simulink model "ClosedLoopControl"  (R2016b)
settings: Solver=FixedStepDiscrete  StartTime=0.0  StopTime=Inf  FixedStep=sCoreParams.core.stepPeriod  RelTol=1e-3  EnableMultiTasking=on
undefined symbols (not defined in the file): fdesignblkfcn, gcbh, High, sCoreParams, sCoreParams_decoders_chanceDetector_randStimEventsPerSec, sCoreParams_decoders_txDetector_channel1, sCoreParams_decoders_txDetector_channel2, sCoreParams_decoders_txDetector_detectChannelInds, sCoreParams_decoders_txDetector_nChannels, sCoreParams_Features_Baseline_initialThresholdValue, sCoreParams_Features_Baseline_weightPreviousThreshold, sCoreParams_Features_Data_SmoothWindowsDurationSamples, sCoreParams_stimulator_stimAfterDelaySteps
libraries: dsparch4 x20, dspstat3 x19, dspspect3 x6, dspfdesign x2, dspindex x2, dspswit3 x1
(part 1 of 6)
settings Model: DataTypeOverride=Double  MinMaxOverflowLogging=ForceOff  Creator=rzelmann  LastModifiedBy=rzelmann
settings SolverCC: EnableConcurrentExecution=on  ConcurrentTasks=on
settings DataIOCC: SaveFormat=StructureWithTime  DSMLogging=off  SignalLoggingName=logsClosedLoopControl
settings OptimizationCC: DefaultParameterBehavior=Inlined  EfficientFloat2IntCast=on  LifeSpan=inf
settings DebuggingCC: AllowSymbolicDim=off  SFUnexpectedBacktrackingDiag=warning  SFNoUnconditionalDefaultTransitionDiag=warning  SFExecutionAtInitializationDiag=none
settings HardwareCC: ProdBitPerPointer=32  ProdBitPerSizeT=32  ProdBitPerPtrDiffT=32  ProdLargestAtomicFloat=None  ProdWordSize=32  ProdLongLongMode=on  ProdHWDeviceType=Generic->32-bit x86 compatible
settings ModelReferenceCC: UpdateModelReferenceTargets=Force  EnableParallelModelReferenceBuilds=on  ParallelModelReferenceMATLABWorkerInit=Copy Base Workspace  ModelReferenceNumInstancesAllowed=Single  ModelReferencePassRootInputsByReference=off
settings RTWCC: SystemTargetFile=slrt.tlc  TemplateMakefile=slrt_default_tmf  Description=Simulink Real-Time  RTWCompilerOptimization=on
settings CodeAppCC: MaxIdLength=63
settings ConfigComp: CovMetricSettings=dw  CovHtmlReporting=on  CovSaveCumulativeToWorkspaceVar=on  CovSaveSingleToWorkspaceVar=on  CovExternalEMLEnable=off

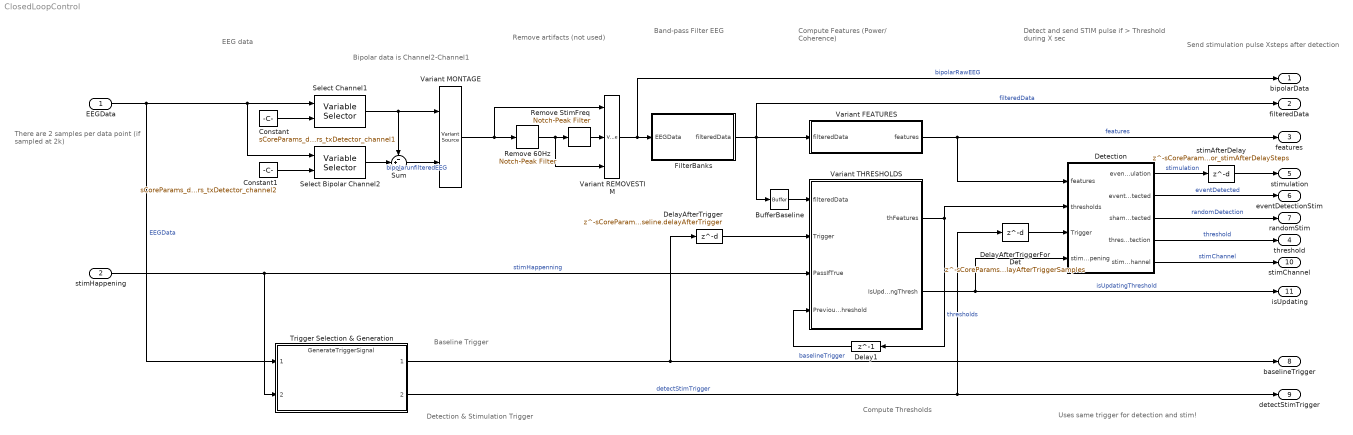
== system ClosedLoopControl ==
  note: Send stimulation pulse Xsteps after detection
  note: Bipolar data is Channel2-Channel1
  note: Baseline Trigger
  note: EEG data
  note: Uses same trigger for detection and stim!
  note: There are 2 samples per data point
      | (if sampled at 2k)
  note: Detection & Stimulation Trigger
  note: Band-pass
      | Filter EEG
  note: Compute Features
      | (Power/ Coherence)
  note: Remove artifacts
      | (not used)
  note: Detect and send STIM pulse
      | if > Threshold during X sec
  note: Compute Thresholds
  EEGData : Inport  OutDataTypeStr=double  PortDimensions=[sCoreParams.core.samplesPerStep sCoreParams.core.maxChannelsAllNSPs]  SampleTime=sCoreParams.core.stepPeriod
  stimHappening : Inport  Port=2  OutDataTypeStr=boolean  PortDimensions=1  SampleTime=sCoreParams.core.stepPeriod
  BufferBaseline : Buffer  N=sCoreParams.Features.Baseline.durationSamples  V=sCoreParams.Features.Baseline.durationSamples-sCoreParams.FrameSize  TreatMby1Signals=One channel  OutputFrames=off
  Constant : Constant  Value=sCoreParams_decoders_txDetector_channel1  SampleTime=Inf
  Constant1 : Constant  Value=sCoreParams_decoders_txDetector_channel2
  Delay1 : Delay  DelayLength=1  InitialCondition=sCoreParams_Features_Baseline_initialThresholdValue  InputProcessing=Inherited  SampleTime=sCoreParams.core.stepPeriod
  DelayAfterTrigger : Delay  DelayLength=sCoreParams.Features.Baseline.delayAfterTrigger  InitialCondition=sCoreParams.Features.Baseline.beforeFirstTrigger  InputProcessing=Columns as channels (frame based)  SampleTime=sCoreParams.core.stepPeriod
  DelayAfterTriggerForDet : Delay  DelayLength=sCoreParams.decoders.txDetector.delayAfterTriggerSamples  InitialCondition=0  InputProcessing=Columns as channels (frame based)  SampleTime=sCoreParams.core.stepPeriod
  Detection : Subsystem
  FilterBanks : Subsystem
  Remove 60Hz : dspfdesign/Notch-Peak Filter  Specification=Bandwidth and center frequency  Bandwidth=2  QualityFactor=5  CenterFrequency=60  BandwidthCoefficient=0.72654  CenterFrequencyCoefficient=0  Output=Notch  InheritSampleRate=off  SampleRate=sCoreParams.core.samplingRate  SimulateUsing=Code generation
  Remove StimFreq : dspfdesign/Notch-Peak Filter  Specification=Bandwidth and center frequency  Bandwidth=2  QualityFactor=5  CenterFrequency=sCoreParams_stimulationFrequencyHz  BandwidthCoefficient=0.72654  CenterFrequencyCoefficient=0  Output=Notch  InheritSampleRate=off  SampleRate=sCoreParams.core.samplingRate  SimulateUsing=Code generation
  Select Bipolar Channel2 : dspindex/Variable Selector  NumInputs=1  rowsOrCols=Columns  IdxMode=Variable  Elements=sCoreParams_decoders_txDetector_channel2  ZerOneIdxMode=One-based  errmode=Clip Index  FillMode=off  FillValues=0
  Select Channel1 : dspindex/Variable Selector  NumInputs=1  rowsOrCols=Columns  IdxMode=Variable  Elements=sCoreParams_decoders_txDetector_channel1  ZerOneIdxMode=One-based  errmode=Clip Index  FillMode=off  FillValues=0
  Sum : Sum  Inputs=-+|  InputSameDT=on
  Trigger Selection & Generation : ModelReference  ModelNameDialog=GenerateTriggerSignal  SimulationMode=Normal  ModelReferenceVersion=1.53
  Variant FEATURES : Subsystem  Variant=on
  Variant MONTAGE : VariantSource  Description=|
      | Variant MONTAGE allows to select between referential and bipolar montages,
      | Output is N referential or bipolar channels.
      | channel numbers are specified in variables:
      |  - sCoreParams.decoders.txDetector.channel1 
      |  - sCoreParams.decoders.txDetector.channel2
      | 
      | In the case of referential only sCoreParams.decoders.txDetector.channel1 is considered
  Variant REMOVESTIM : VariantSource  Description=|
      | Variant MONTAGE allows to select between referential and bipolar montages,
      | Output is N referential or bipolar channels.
      | channel numbers are specified in variables:
      |  - sCoreParams.decoders.txDetector.channel1 
      |  - sCoreParams.decoders.txDetector.channel2
      | 
      | In the case of referential only sCoreParams.decoders.txDetector.channel1 is considered
  Variant THRESHOLDS : Subsystem  Variant=on
  stimAfterDelay : Delay  DelayLength=sCoreParams_stimulator_stimAfterDelaySteps  InitialCondition=0  InputProcessing=Columns as channels (frame based)  SampleTime=sCoreParams.core.stepPeriod
  bipolarData : Outport
  filteredData : Outport  Port=2
  features : Outport  Port=3  SampleTime=sCoreParams.core.stepPeriod  BusOutputAsStruct=on
  threshold : Outport  Port=4
  stimulation : Outport  Port=5
  eventDetectionStim : Outport  Port=6
  randomStim : Outport  Port=7  OutDataTypeStr=boolean
  baselineTrigger : Outport  Port=8
  detectStimTrigger : Outport  Port=9
  stimChannel : Outport  Port=10  OutDataTypeStr=int32  PortDimensions=[1 2]
  isUpdating : Outport  Port=11
  wires:
  Detection/4(thresholdUsedInDetection) -> threshold/1  "threshold"
  Variant MONTAGE/1 -> Variant REMOVESTIM/1, Remove 60Hz/1
  Variant THRESHOLDS/2(IsUpdatingThresh) -> Detection/4(stimHappening), isUpdating/1  "isUpdatingThreshold"
  Select Channel1/1 -> Variant MONTAGE/1, Sum/1
  Sum/1 -> Variant MONTAGE/2  "bipolarunfilteredEEG"
  Select Bipolar Channel2/1 -> Sum/2
  Trigger Selection & Generation/1 -> DelayAfterTrigger/1, baselineTrigger/1  "baselineTrigger"
  Remove 60Hz/1 -> Variant REMOVESTIM/3, Remove StimFreq/1
  Variant REMOVESTIM/1 -> FilterBanks/1(EEGData), bipolarData/1  "bipolarRawEEG"
  stimHappening/1 -> Trigger Selection & Generation/2, Variant THRESHOLDS/3(PassIfTrue)  "stimHappenning"
  Constant/1 -> Select Channel1/2
  Constant1/1 -> Select Bipolar Channel2/2
  BufferBaseline/1 -> Variant THRESHOLDS/1(filteredData)
  Variant FEATURES/1(features) -> Detection/1(features), features/1  "features"
  Variant THRESHOLDS/1(thFeatures) -> Delay1/1, Detection/2(thresholds)  "thresholds"
  Delay1/1 -> Variant THRESHOLDS/4(PreviousThreshold)
  DelayAfterTrigger/1 -> Variant THRESHOLDS/2(Trigger)
  Trigger Selection & Generation/2 -> DelayAfterTriggerForDet/1, detectStimTrigger/1  "detectStimTrigger"
  DelayAfterTriggerForDet/1 -> Detection/3(Trigger)
  Detection/5(stimChannel) -> stimChannel/1  "stimChannel"
  EEGData/1 -> Select Bipolar Channel2/1, Select Channel1/1, Trigger Selection & Generation/1  "EEGData"
  Remove StimFreq/1 -> Variant REMOVESTIM/2
  FilterBanks/1(filteredData) -> BufferBaseline/1, filteredData/1, Variant FEATURES/1(filteredData)  "filteredData"
  Detection/3(shamDetected) -> randomStim/1  "randomDetection"
  Detection/2(eventDetected) -> eventDetectionStim/1  "eventDetected"
  Detection/1(eventStimulation) -> stimAfterDelay/1  "stimulation"
  stimAfterDelay/1 -> stimulation/1

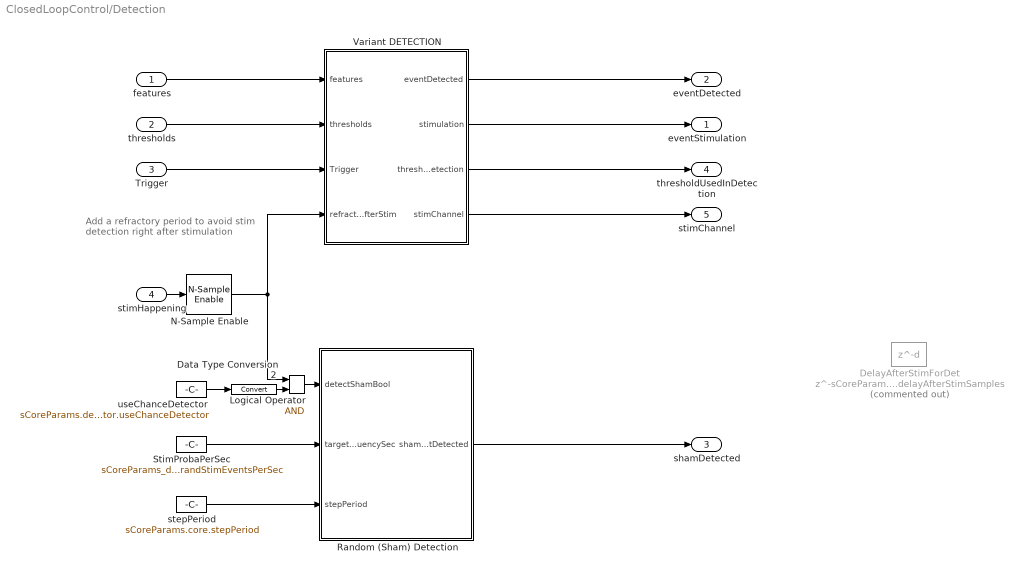
== system ClosedLoopControl/Detection ==
  note: Add a refractory period to avoid
      | stim detection right after stimulation
  features : Inport
  thresholds : Inport  Port=2
  Trigger : Inport  Port=3
  stimHappening : Inport  Port=4
  Data Type Conversion2 : DataTypeConversion
  DelayAfterStimForDet : Delay  Commented=on  DelayLength=sCoreParams.decoders.txDetector.delayAfterStimSamples  InitialCondition=0  InputProcessing=Columns as channels (frame based)  SampleTime=sCoreParams.core.stepPeriod
  Logical Operator : Logic  IconShape=distinctive  AllPortsSameDT=off  OutDataTypeStr=boolean
  N-Sample Enable : dspswit3/N-Sample Enable  N=sCoreParams.decoders.txDetector.delayAfterStimSteps  ActiveLevel=High (1)  reset=on  TriggerType=Rising edge  Ts=1  DataType=Logical
  Random (Sham) Detection : MATLAB Function  TreatAsAtomicUnit=on  SystemSampleTime=sCoreParams.core.stepPeriod
  StimProbaPerSec : Constant  Value=sCoreParams_decoders_chanceDetector_randStimEventsPerSec
  Variant DETECTION : Subsystem  Variant=on
  stepPeriod : Constant  Value=sCoreParams.core.stepPeriod
  useChanceDetector : Constant  Value=sCoreParams.decoders.chanceDetector.useChanceDetector
  eventStimulation : Outport
  eventDetected : Outport  Port=2
  shamDetected : Outport  Port=3  OutDataTypeStr=boolean
  thresholdUsedInDetection : Outport  Port=4
  stimChannel : Outport  Port=5
  wires:
  Variant DETECTION/2(stimulation) -> eventStimulation/1
  features/1 -> Variant DETECTION/1(features)
  thresholds/1 -> Variant DETECTION/2(thresholds)
  Trigger/1 -> Variant DETECTION/3(Trigger)
  Variant DETECTION/3(thresholdUsedInDetection) -> thresholdUsedInDetection/1
  Variant DETECTION/4(stimChannel) -> stimChannel/1
  stepPeriod/1 -> Random (Sham) Detection/3(stepPeriod)
  StimProbaPerSec/1 -> Random (Sham) Detection/2(targetShamFrequencySec)
  Logical Operator/1 -> Random (Sham) Detection/1(detectShamBool)
  Random (Sham) Detection/1(shamEventDetected) -> shamDetected/1
  Variant DETECTION/1(eventDetected) -> eventDetected/1
  stimHappening/1 -> N-Sample Enable/1
  N-Sample Enable/1 -> Logical Operator/1, Variant DETECTION/4(refractoryTimeAfterStim)
  useChanceDetector/1 -> Data Type Conversion2/1
  Data Type Conversion2/1 -> Logical Operator/2

== system ClosedLoopControl/FilterBanks ==
  note: Frequency band of the filter is FIXED in Simulink Real-Time
      | Add a new variant block if other sampling rates are required
  EEGData : Inport
  Variant FILTER 1000 : Subsystem  Variant=on
  Variant FILTER 2000 : Subsystem  Variant=on
  Variant SAMPLING RATE : VariantSource  Description=|
      | Variant MONTAGE allows to select between referential and bipolar montages,
      | Output is N referential or bipolar channels.
      | channel numbers are specified in variables:
      |  - sCoreParams.decoders.txDetector.channel1 
      |  - sCoreParams.decoders.txDetector.channel2
      | 
      | In the case of referential only sCoreParams.decoders.txDetector.channel1 is considered
  filteredData : Outport
  wires:
  Variant FILTER 1000/1(filteredData) -> Variant SAMPLING RATE/1  "filteredData1000"
  EEGData/1 -> Variant FILTER 1000/1(EEGData), Variant FILTER 2000/1(EEGData)
  Variant FILTER 2000/1(filteredData) -> Variant SAMPLING RATE/2  "filteredData2000"
  Variant SAMPLING RATE/1 -> filteredData/1  "filteredData"

== system ClosedLoopControl/Variant FEATURES ==
  note: 1) Add Subsystem or Model blocks as valid variant choices.
      | 2) You cannot connect blocks at this level. At simulation, connectivity is automatically
      | determined, based on the active variant and port name matching.
  filteredData : Inport  SampleTime=sCoreParams.core.stepPeriod
  BandPower : Subsystem  TreatAsAtomicUnit=on  SystemSampleTime=sCoreParams.core.stepPeriod  VariantControl=variantParams_FEATURE_BANDPOWER
  BandPowerSmooth : Subsystem  TreatAsAtomicUnit=on  SystemSampleTime=sCoreParams.core.stepPeriod  VariantControl=variantParams_FEATURE_SMOOTHBANDPOWER
  Coherence : ModelReference  ModelNameDialog=ComputeCoherence.slx  VariantControl=variantParams_FEATURE_COHERENCE  ModelReferenceVersion=1.18
  Correlation : Subsystem  TreatAsAtomicUnit=on  SystemSampleTime=sCoreParams.core.stepPeriod  VariantControl=variantParams_FEATURE_CORRELATION
  Variance : Subsystem  TreatAsAtomicUnit=on  SystemSampleTime=sCoreParams.core.stepPeriod  VariantControl=variantParams_FEATURE_VARIANCE
  VarianceOfPower : Subsystem  TreatAsAtomicUnit=on  SystemSampleTime=sCoreParams.core.stepPeriod  VariantControl=variantParams_FEATURE_VARIANCEOFPOWER
  features : Outport  SampleTime=sCoreParams.core.stepPeriod

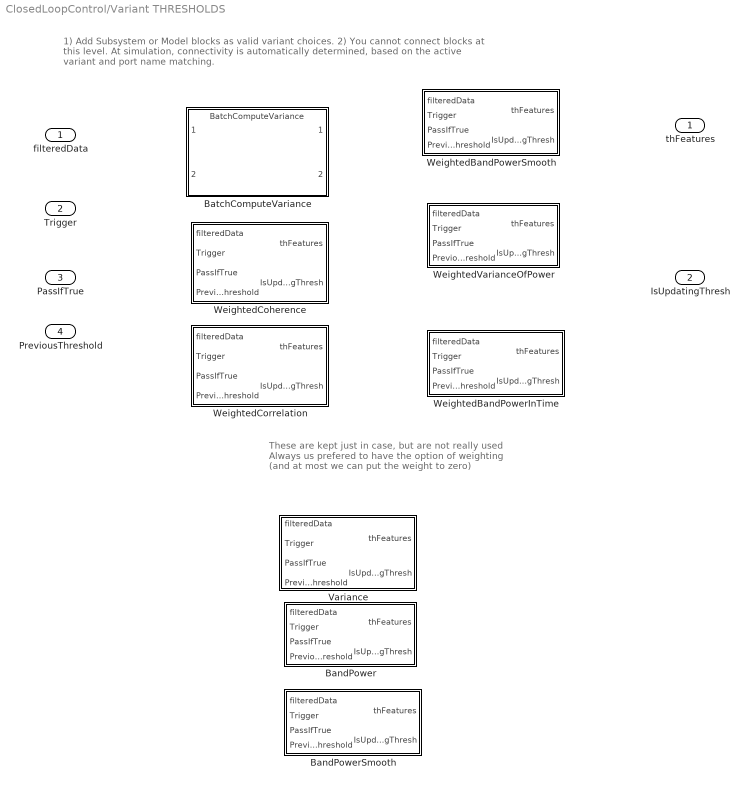
== system ClosedLoopControl/Variant THRESHOLDS ==
  note: These are kept just in case, but are not really used
      | Always us prefered to have the option of weighting
      | (and at most we can put the weight to zero)
  note: 1) Add Subsystem or Model blocks as valid variant choices.
      | 2) You cannot connect blocks at this level. At simulation, connectivity is automatically
      | determined, based on the active variant and port name matching.
  filteredData : Inport  SampleTime=sCoreParams.core.stepPeriod
  Trigger : Inport  Port=2  SampleTime=sCoreParams.core.stepPeriod
  PassIfTrue : Inport  Port=3  OutDataTypeStr=boolean  SampleTime=sCoreParams.core.stepPeriod
  PreviousThreshold : Inport  Port=4  SampleTime=sCoreParams.core.stepPeriod
  BandPower : Subsystem  TreatAsAtomicUnit=on  SystemSampleTime=sCoreParams.core.stepPeriod  VariantControl=variantParams_FEATURE_BASELINE_BANDPOWER
  BandPowerSmooth : Subsystem  TreatAsAtomicUnit=on  SystemSampleTime=sCoreParams.core.stepPeriod  VariantControl=variantParams_FEATURE_BASELINE_SMOOTHBANDPOWER
  BatchComputeVariance : ModelReference  ModelNameDialog=BatchComputeVariance  SimulationMode=Normal  VariantControl=variantParams_FEATURE_BASELINE_BATCHVARIANCE  ModelReferenceVersion=1.126
  Variance : Subsystem  TreatAsAtomicUnit=on  SystemSampleTime=sCoreParams.core.stepPeriod  VariantControl=variantParams_FEATURE_BASELINE_VARIANCE
  WeightedBandPowerInTime : Subsystem  TreatAsAtomicUnit=on  SystemSampleTime=sCoreParams.core.stepPeriod  VariantControl=variantParams_FEATURE_BASELINE_WEIGHTEDTIMEPOWER
  WeightedBandPowerSmooth : Subsystem  TreatAsAtomicUnit=on  SystemSampleTime=sCoreParams.core.stepPeriod  VariantControl=variantParams_FEATURE_BASELINE_WEIGHTEDPOWER
  WeightedCoherence : Subsystem  TreatAsAtomicUnit=on  SystemSampleTime=sCoreParams.core.stepPeriod  VariantControl=variantParams_FEATURE_BASELINE_COHERENCE
  WeightedCorrelation : Subsystem  TreatAsAtomicUnit=on  SystemSampleTime=sCoreParams.core.stepPeriod  VariantControl=variantParams_FEATURE_BASELINE_CORRELATION
  WeightedVarianceOfPower : Subsystem  TreatAsAtomicUnit=on  SystemSampleTime=sCoreParams.core.stepPeriod  VariantControl=variantParams_FEATURE_BASELINE_VARIANCEOFPOWER
  thFeatures : Outport  SampleTime=sCoreParams.core.stepPeriod
  IsUpdatingThresh : Outport  Port=2  SampleTime=sCoreParams.core.stepPeriod

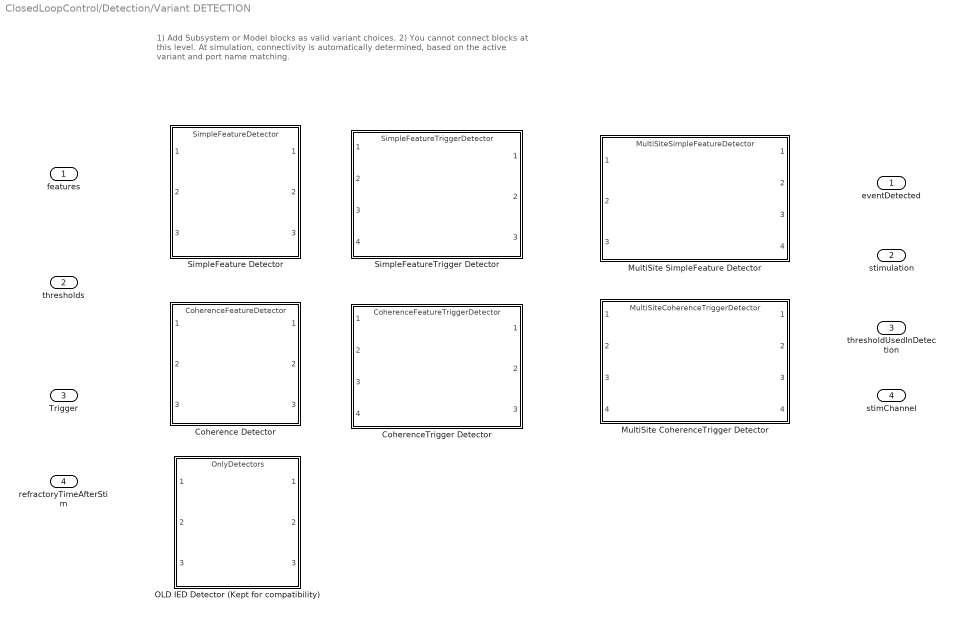
== system ClosedLoopControl/Detection/Variant DETECTION ==
  note: 1) Add Subsystem or Model blocks as valid variant choices.
      | 2) You cannot connect blocks at this level. At simulation, connectivity is automatically
      | determined, based on the active variant and port name matching.
  features : Inport
  thresholds : Inport  Port=2
  Trigger : Inport  Port=3
  refractoryTimeAfterStim : Inport  Port=4
  Coherence Detector : ModelReference  ModelNameDialog=CoherenceFeatureDetector.slx  SimulationMode=Normal  VariantControl=variantParams_DETECTOR_COHERENCEFEATURE  ModelReferenceVersion=1.310
  CoherenceTrigger Detector : ModelReference  ModelNameDialog=CoherenceFeatureTriggerDetector.slx  SimulationMode=Normal  VariantControl=variantParams_DETECTOR_COHERENCEFEATURETRIGGER  ModelReferenceVersion=1.317
  MultiSite CoherenceTrigger Detector : ModelReference  ModelNameDialog=MultiSiteCoherenceTriggerDetector.slx  SimulationMode=Normal  VariantControl=variantParams_DETECTOR_MULTISITECOHERENCETRIGGER  ModelReferenceVersion=1.341
  MultiSite SimpleFeature Detector : ModelReference  ModelNameDialog=MultiSiteSimpleFeatureDetector.slx  SimulationMode=Normal  VariantControl=variantParams_DETECTOR_MULTISITESIMPLEFEATURE  ModelReferenceVersion=1.305
  OLD IED Detector (Kept for compatibility) : ModelReference  ModelNameDialog=OnlyDetectors  SimulationMode=Normal  VariantControl=variantParams_DETECTOR_IED  ModelReferenceVersion=1.253
  SimpleFeature Detector : ModelReference  ModelNameDialog=SimpleFeatureDetector.slx  SimulationMode=Normal  VariantControl=variantParams_DETECTOR_SIMPLEFEATURE  ModelReferenceVersion=1.312
  SimpleFeatureTrigger Detector : ModelReference  ModelNameDialog=SimpleFeatureTriggerDetector.slx  SimulationMode=Normal  VariantControl=variantParams_DETECTOR_SIMPLEFEATURETRIGGER  ModelReferenceVersion=1.312
  eventDetected : Outport
  stimulation : Outport  Port=2
  thresholdUsedInDetection : Outport  Port=3
  stimChannel : Outport  Port=4

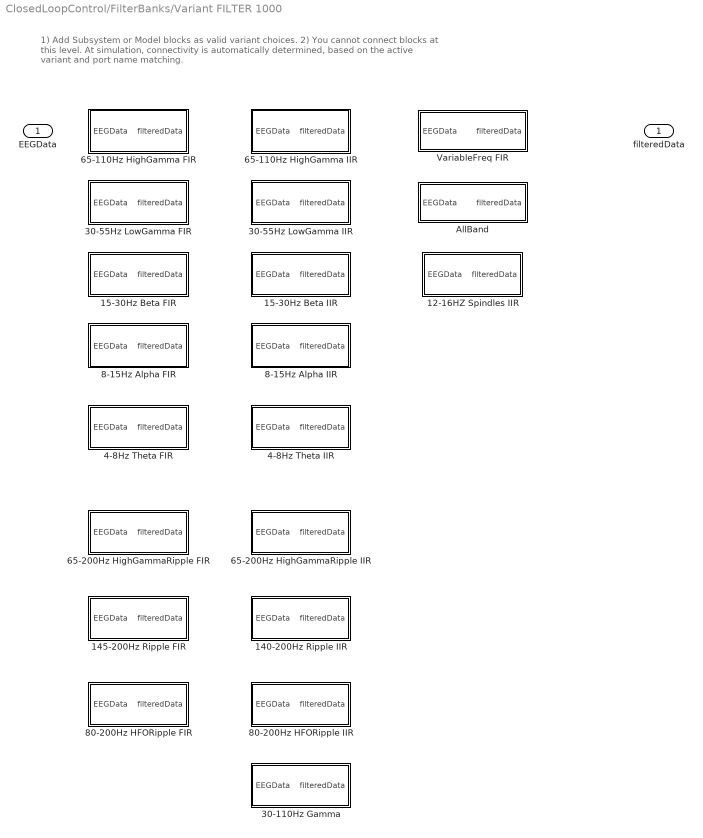
== system ClosedLoopControl/FilterBanks/Variant FILTER 1000 ==
  note: 1) Add Subsystem or Model blocks as valid variant choices.
      | 2) You cannot connect blocks at this level. At simulation, connectivity is automatically
      | determined, based on the active variant and port name matching.
  EEGData : Inport  SampleTime=sCoreParams.core.stepPeriod
  12-16HZ Spindles IIR : Subsystem  DialogController=fdesignblkfcn  InitFcn=fdesignblkfcn(gcbh, {'InitFcn'});  TreatAsAtomicUnit=on  SystemSampleTime=sCoreParams.core.stepPeriod  VariantControl=variantParams_FILTER_IIR_SPINDLES  mask(Bandpass Filter){}
      mask help: Design a bandpass filter
      settings: CopyFcn=fdesignblkfcn(gcbh, {'CopyFcn'});
      mask Help: helpview(mapfilelocation('dsp'), 'dspbandpassfilter');
      mask Display: disp('Bandpass');
  140-200Hz Ripple IIR : Subsystem  DialogController=fdesignblkfcn  InitFcn=fdesignblkfcn(gcbh, {'InitFcn'});  TreatAsAtomicUnit=on  SystemSampleTime=sCoreParams.core.stepPeriod  VariantControl=variantParams_FILTER_IIR_RIPPLE  mask(Bandpass Filter){}
      mask help: Design a bandpass filter
      settings: CopyFcn=fdesignblkfcn(gcbh, {'CopyFcn'});
      mask Help: helpview(mapfilelocation('dsp'), 'dspbandpassfilter');
      mask Display: disp('Bandpass');
  145-200Hz Ripple FIR : Subsystem  DialogController=fdesignblkfcn  InitFcn=fdesignblkfcn(gcbh, {'InitFcn'});  TreatAsAtomicUnit=on  SystemSampleTime=sCoreParams.core.stepPeriod  VariantControl=variantParams_FILTER_FIR_RIPPLE  mask(Bandpass Filter){}
      mask help: Design a bandpass filter
      settings: CopyFcn=fdesignblkfcn(gcbh, {'CopyFcn'});
      mask Help: helpview(mapfilelocation('dsp'), 'dspbandpassfilter');
      mask Display: disp('Bandpass');
  15-30Hz Beta FIR : Subsystem  DialogController=fdesignblkfcn  InitFcn=fdesignblkfcn(gcbh, {'InitFcn'});  TreatAsAtomicUnit=on  SystemSampleTime=sCoreParams.core.stepPeriod  VariantControl=variantParams_FILTER_FIR_BETA  mask(Bandpass Filter){}
      mask help: Design a bandpass filter
      settings: CopyFcn=fdesignblkfcn(gcbh, {'CopyFcn'});
      mask Help: helpview(mapfilelocation('dsp'), 'dspbandpassfilter');
      mask Display: disp('Bandpass');
  15-30Hz Beta IIR : Subsystem  DialogController=fdesignblkfcn  InitFcn=fdesignblkfcn(gcbh, {'InitFcn'});  TreatAsAtomicUnit=on  SystemSampleTime=sCoreParams.core.stepPeriod  VariantControl=variantParams_FILTER_IIR_BETA  mask(Bandpass Filter){}
      mask help: Design a bandpass filter
      settings: CopyFcn=fdesignblkfcn(gcbh, {'CopyFcn'});
      mask Help: helpview(mapfilelocation('dsp'), 'dspbandpassfilter');
      mask Display: disp('Bandpass');
  30-110Hz Gamma : Subsystem  DialogController=fdesignblkfcn  InitFcn=fdesignblkfcn(gcbh, {'InitFcn'});  TreatAsAtomicUnit=on  SystemSampleTime=sCoreParams.core.stepPeriod  VariantControl=variantParams_FILTER_IIR_GAMMA  mask(Bandpass Filter){}
      mask help: Design a bandpass filter
      settings: CopyFcn=fdesignblkfcn(gcbh, {'CopyFcn'});
      mask Help: helpview(mapfilelocation('dsp'), 'dspbandpassfilter');
      mask Display: disp('Bandpass');
  30-55Hz LowGamma FIR : Subsystem  DialogController=fdesignblkfcn  InitFcn=fdesignblkfcn(gcbh, {'InitFcn'});  TreatAsAtomicUnit=on  SystemSampleTime=sCoreParams.core.stepPeriod  VariantControl=variantParams_FILTER_FIR_LOWGAMMA  mask(Bandpass Filter){}
      mask help: Design a bandpass filter
      settings: CopyFcn=fdesignblkfcn(gcbh, {'CopyFcn'});
      mask Help: helpview(mapfilelocation('dsp'), 'dspbandpassfilter');
      mask Display: disp('Bandpass');
  30-55Hz LowGamma IIR : Subsystem  DialogController=fdesignblkfcn  InitFcn=fdesignblkfcn(gcbh, {'InitFcn'});  TreatAsAtomicUnit=on  SystemSampleTime=sCoreParams.core.stepPeriod  VariantControl=variantParams_FILTER_IIR_LOWGAMMA  mask(Bandpass Filter){}
      mask help: Design a bandpass filter
      settings: CopyFcn=fdesignblkfcn(gcbh, {'CopyFcn'});
      mask Help: helpview(mapfilelocation('dsp'), 'dspbandpassfilter');
      mask Display: disp('Bandpass');
  4-8Hz Theta FIR : Subsystem  DialogController=fdesignblkfcn  InitFcn=fdesignblkfcn(gcbh, {'InitFcn'});  TreatAsAtomicUnit=on  SystemSampleTime=sCoreParams.core.stepPeriod  VariantControl=variantParams_FILTER_FIR_THETA  mask(Bandpass Filter){}
      mask help: Design a bandpass filter
      settings: CopyFcn=fdesignblkfcn(gcbh, {'CopyFcn'});
      mask Help: helpview(mapfilelocation('dsp'), 'dspbandpassfilter');
      mask Display: disp('Bandpass');
  4-8Hz Theta IIR : Subsystem  DialogController=fdesignblkfcn  InitFcn=fdesignblkfcn(gcbh, {'InitFcn'});  TreatAsAtomicUnit=on  SystemSampleTime=sCoreParams.core.stepPeriod  VariantControl=variantParams_FILTER_IIR_THETA  mask(Bandpass Filter){}
      mask help: Design a bandpass filter
      settings: CopyFcn=fdesignblkfcn(gcbh, {'CopyFcn'});
      mask Help: helpview(mapfilelocation('dsp'), 'dspbandpassfilter');
      mask Display: disp('Bandpass');
  65-110Hz HighGamma FIR : Subsystem  DialogController=fdesignblkfcn  InitFcn=fdesignblkfcn(gcbh, {'InitFcn'});  TreatAsAtomicUnit=on  SystemSampleTime=sCoreParams.core.stepPeriod  VariantControl=variantParams_FILTER_FIR_HIGHGAMMA  mask(Bandpass Filter){}
      mask help: Design a bandpass filter
      settings: CopyFcn=fdesignblkfcn(gcbh, {'CopyFcn'});
      mask Help: helpview(mapfilelocation('dsp'), 'dspbandpassfilter');
      mask Display: disp('Bandpass');
  65-110Hz HighGamma IIR : Subsystem  DialogController=fdesignblkfcn  InitFcn=fdesignblkfcn(gcbh, {'InitFcn'});  TreatAsAtomicUnit=on  SystemSampleTime=sCoreParams.core.stepPeriod  VariantControl=variantParams_FILTER_IIR_HIGHGAMMA  mask(Bandpass Filter){}
      mask help: Design a bandpass filter
      settings: CopyFcn=fdesignblkfcn(gcbh, {'CopyFcn'});
      mask Help: helpview(mapfilelocation('dsp'), 'dspbandpassfilter');
      mask Display: disp('Bandpass');
  65-200Hz HighGammaRipple FIR : Subsystem  DialogController=fdesignblkfcn  InitFcn=fdesignblkfcn(gcbh, {'InitFcn'});  TreatAsAtomicUnit=on  SystemSampleTime=sCoreParams.core.stepPeriod  VariantControl=variantParams_FILTER_FIR_HIGHGAMMARIPPLE  mask(Bandpass Filter){}
      mask help: Design a bandpass filter
      settings: CopyFcn=fdesignblkfcn(gcbh, {'CopyFcn'});
      mask Help: helpview(mapfilelocation('dsp'), 'dspbandpassfilter');
      mask Display: disp('Bandpass');
  65-200Hz HighGammaRipple IIR : Subsystem  DialogController=fdesignblkfcn  InitFcn=fdesignblkfcn(gcbh, {'InitFcn'});  TreatAsAtomicUnit=on  SystemSampleTime=sCoreParams.core.stepPeriod  VariantControl=variantParams_FILTER_IIR_HIGHGAMMARIPPLE  mask(Bandpass Filter){}
      mask help: Design a bandpass filter
      settings: CopyFcn=fdesignblkfcn(gcbh, {'CopyFcn'});
      mask Help: helpview(mapfilelocation('dsp'), 'dspbandpassfilter');
      mask Display: disp('Bandpass');
  8-15Hz Alpha FIR : Subsystem  DialogController=fdesignblkfcn  InitFcn=fdesignblkfcn(gcbh, {'InitFcn'});  TreatAsAtomicUnit=on  SystemSampleTime=sCoreParams.core.stepPeriod  VariantControl=variantParams_FILTER_FIR_ALPHA  mask(Bandpass Filter){}
      mask help: Design a bandpass filter
      settings: CopyFcn=fdesignblkfcn(gcbh, {'CopyFcn'});
      mask Help: helpview(mapfilelocation('dsp'), 'dspbandpassfilter');
      mask Display: disp('Bandpass');
  8-15Hz Alpha IIR : Subsystem  DialogController=fdesignblkfcn  InitFcn=fdesignblkfcn(gcbh, {'InitFcn'});  TreatAsAtomicUnit=on  SystemSampleTime=sCoreParams.core.stepPeriod  VariantControl=variantParams_FILTER_IIR_ALPHA  mask(Bandpass Filter){}
      mask help: Design a bandpass filter
      settings: CopyFcn=fdesignblkfcn(gcbh, {'CopyFcn'});
      mask Help: helpview(mapfilelocation('dsp'), 'dspbandpassfilter');
      mask Display: disp('Bandpass');
  80-200Hz HFORipple FIR : Subsystem  DialogController=fdesignblkfcn  InitFcn=fdesignblkfcn(gcbh, {'InitFcn'});  TreatAsAtomicUnit=on  SystemSampleTime=sCoreParams.core.stepPeriod  VariantControl=variantParams_FILTER_FIR_HFORIPPLE  mask(Bandpass Filter){}
      mask help: Design a bandpass filter
      settings: CopyFcn=fdesignblkfcn(gcbh, {'CopyFcn'});
      mask Help: helpview(mapfilelocation('dsp'), 'dspbandpassfilter');
      mask Display: disp('Bandpass');
  80-200Hz HFORipple IIR : Subsystem  DialogController=fdesignblkfcn  InitFcn=fdesignblkfcn(gcbh, {'InitFcn'});  TreatAsAtomicUnit=on  SystemSampleTime=sCoreParams.core.stepPeriod  VariantControl=variantParams_FILTER_IIR_HFORIPPLE  mask(Bandpass Filter){}
      mask help: Design a bandpass filter
      settings: CopyFcn=fdesignblkfcn(gcbh, {'CopyFcn'});
      mask Help: helpview(mapfilelocation('dsp'), 'dspbandpassfilter');
      mask Display: disp('Bandpass');
  AllBand : Subsystem  TreatAsAtomicUnit=on  SystemSampleTime=sCoreParams.core.stepPeriod  VariantControl=variantParams_FILTER_ALLPASS
  VariableFreq FIR : Subsystem  TreatAsAtomicUnit=on  SystemSampleTime=sCoreParams.core.stepPeriod  VariantControl=variantParams_FILTER_FIR_EXTERNAL
  filteredData : Outport  SampleTime=sCoreParams.core.stepPeriod

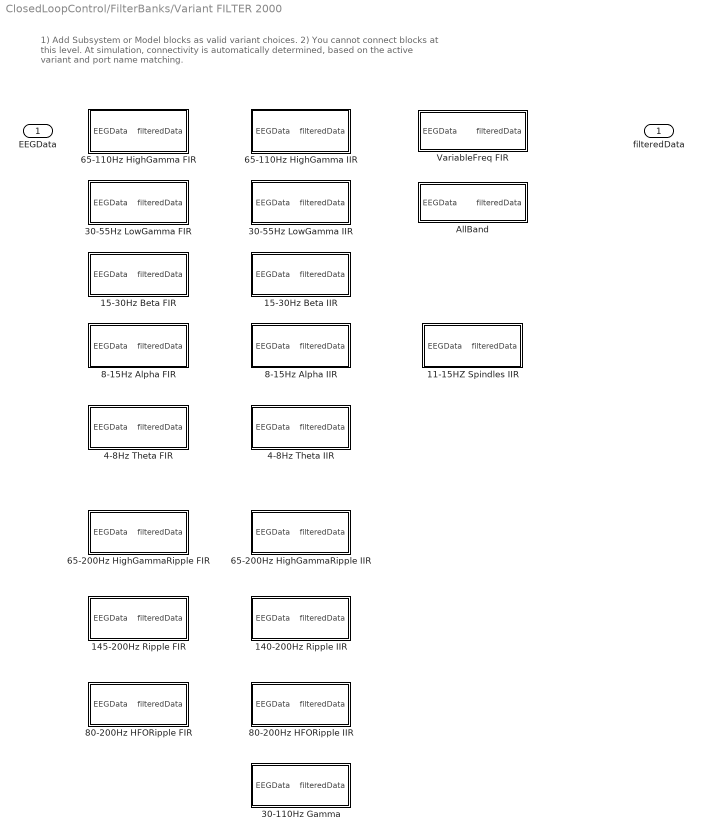
== system ClosedLoopControl/FilterBanks/Variant FILTER 2000 ==
  note: 1) Add Subsystem or Model blocks as valid variant choices.
      | 2) You cannot connect blocks at this level. At simulation, connectivity is automatically
      | determined, based on the active variant and port name matching.
  EEGData : Inport  SampleTime=sCoreParams.core.stepPeriod
  11-15HZ Spindles IIR : Subsystem  DialogController=fdesignblkfcn  InitFcn=fdesignblkfcn(gcbh, {'InitFcn'});  TreatAsAtomicUnit=on  SystemSampleTime=sCoreParams.core.stepPeriod  VariantControl=variantParams_FILTER_IIR_SPINDLES  mask(Bandpass Filter){}
      mask help: Design a bandpass filter
      settings: CopyFcn=fdesignblkfcn(gcbh, {'CopyFcn'});
      mask Help: helpview(mapfilelocation('dsp'), 'dspbandpassfilter');
      mask Display: disp('Bandpass');
  140-200Hz Ripple IIR : Subsystem  DialogController=fdesignblkfcn  InitFcn=fdesignblkfcn(gcbh, {'InitFcn'});  TreatAsAtomicUnit=on  SystemSampleTime=sCoreParams.core.stepPeriod  VariantControl=variantParams_FILTER_IIR_RIPPLE  mask(Bandpass Filter){}
      mask help: Design a bandpass filter
      settings: CopyFcn=fdesignblkfcn(gcbh, {'CopyFcn'});
      mask Help: helpview(mapfilelocation('dsp'), 'dspbandpassfilter');
      mask Display: disp('Bandpass');
  145-200Hz Ripple FIR : Subsystem  DialogController=fdesignblkfcn  InitFcn=fdesignblkfcn(gcbh, {'InitFcn'});  TreatAsAtomicUnit=on  SystemSampleTime=sCoreParams.core.stepPeriod  VariantControl=variantParams_FILTER_FIR_RIPPLE  mask(Bandpass Filter){}
      mask help: Design a bandpass filter
      settings: CopyFcn=fdesignblkfcn(gcbh, {'CopyFcn'});
      mask Help: helpview(mapfilelocation('dsp'), 'dspbandpassfilter');
      mask Display: disp('Bandpass');
  15-30Hz Beta FIR : Subsystem  DialogController=fdesignblkfcn  InitFcn=fdesignblkfcn(gcbh, {'InitFcn'});  TreatAsAtomicUnit=on  SystemSampleTime=sCoreParams.core.stepPeriod  VariantControl=variantParams_FILTER_FIR_BETA  mask(Bandpass Filter){}
      mask help: Design a bandpass filter
      settings: CopyFcn=fdesignblkfcn(gcbh, {'CopyFcn'});
      mask Help: helpview(mapfilelocation('dsp'), 'dspbandpassfilter');
      mask Display: disp('Bandpass');
  15-30Hz Beta IIR : Subsystem  DialogController=fdesignblkfcn  InitFcn=fdesignblkfcn(gcbh, {'InitFcn'});  TreatAsAtomicUnit=on  SystemSampleTime=sCoreParams.core.stepPeriod  VariantControl=variantParams_FILTER_IIR_BETA  mask(Bandpass Filter){}
      mask help: Design a bandpass filter
      settings: CopyFcn=fdesignblkfcn(gcbh, {'CopyFcn'});
      mask Help: helpview(mapfilelocation('dsp'), 'dspbandpassfilter');
      mask Display: disp('Bandpass');
  30-110Hz Gamma : Subsystem  DialogController=fdesignblkfcn  InitFcn=fdesignblkfcn(gcbh, {'InitFcn'});  TreatAsAtomicUnit=on  SystemSampleTime=sCoreParams.core.stepPeriod  VariantControl=variantParams_FILTER_IIR_GAMMA  mask(Bandpass Filter){}
      mask help: Design a bandpass filter
      settings: CopyFcn=fdesignblkfcn(gcbh, {'CopyFcn'});
      mask Help: helpview(mapfilelocation('dsp'), 'dspbandpassfilter');
      mask Display: disp('Bandpass');
  30-55Hz LowGamma FIR : Subsystem  DialogController=fdesignblkfcn  InitFcn=fdesignblkfcn(gcbh, {'InitFcn'});  TreatAsAtomicUnit=on  SystemSampleTime=sCoreParams.core.stepPeriod  VariantControl=variantParams_FILTER_FIR_LOWGAMMA  mask(Bandpass Filter){}
      mask help: Design a bandpass filter
      settings: CopyFcn=fdesignblkfcn(gcbh, {'CopyFcn'});
      mask Help: helpview(mapfilelocation('dsp'), 'dspbandpassfilter');
      mask Display: disp('Bandpass');
  30-55Hz LowGamma IIR : Subsystem  DialogController=fdesignblkfcn  InitFcn=fdesignblkfcn(gcbh, {'InitFcn'});  TreatAsAtomicUnit=on  SystemSampleTime=sCoreParams.core.stepPeriod  VariantControl=variantParams_FILTER_IIR_LOWGAMMA  mask(Bandpass Filter){}
      mask help: Design a bandpass filter
      settings: CopyFcn=fdesignblkfcn(gcbh, {'CopyFcn'});
      mask Help: helpview(mapfilelocation('dsp'), 'dspbandpassfilter');
      mask Display: disp('Bandpass');
  4-8Hz Theta FIR : Subsystem  DialogController=fdesignblkfcn  InitFcn=fdesignblkfcn(gcbh, {'InitFcn'});  TreatAsAtomicUnit=on  SystemSampleTime=sCoreParams.core.stepPeriod  VariantControl=variantParams_FILTER_FIR_THETA  mask(Bandpass Filter){}
      mask help: Design a bandpass filter
      settings: CopyFcn=fdesignblkfcn(gcbh, {'CopyFcn'});
      mask Help: helpview(mapfilelocation('dsp'), 'dspbandpassfilter');
      mask Display: disp('Bandpass');
  4-8Hz Theta IIR : Subsystem  DialogController=fdesignblkfcn  InitFcn=fdesignblkfcn(gcbh, {'InitFcn'});  TreatAsAtomicUnit=on  SystemSampleTime=sCoreParams.core.stepPeriod  VariantControl=variantParams_FILTER_IIR_THETA  mask(Bandpass Filter){}
      mask help: Design a bandpass filter
      settings: CopyFcn=fdesignblkfcn(gcbh, {'CopyFcn'});
      mask Help: helpview(mapfilelocation('dsp'), 'dspbandpassfilter');
      mask Display: disp('Bandpass');
  65-110Hz HighGamma FIR : Subsystem  DialogController=fdesignblkfcn  InitFcn=fdesignblkfcn(gcbh, {'InitFcn'});  TreatAsAtomicUnit=on  SystemSampleTime=sCoreParams.core.stepPeriod  VariantControl=variantParams_FILTER_FIR_HIGHGAMMA  mask(Bandpass Filter){}
      mask help: Design a bandpass filter
      settings: CopyFcn=fdesignblkfcn(gcbh, {'CopyFcn'});
      mask Help: helpview(mapfilelocation('dsp'), 'dspbandpassfilter');
      mask Display: disp('Bandpass');
  65-110Hz HighGamma IIR : Subsystem  DialogController=fdesignblkfcn  InitFcn=fdesignblkfcn(gcbh, {'InitFcn'});  TreatAsAtomicUnit=on  SystemSampleTime=sCoreParams.core.stepPeriod  VariantControl=variantParams_FILTER_IIR_HIGHGAMMA  mask(Bandpass Filter){}
      mask help: Design a bandpass filter
      settings: CopyFcn=fdesignblkfcn(gcbh, {'CopyFcn'});
      mask Help: helpview(mapfilelocation('dsp'), 'dspbandpassfilter');
      mask Display: disp('Bandpass');
  65-200Hz HighGammaRipple FIR : Subsystem  DialogController=fdesignblkfcn  InitFcn=fdesignblkfcn(gcbh, {'InitFcn'});  TreatAsAtomicUnit=on  SystemSampleTime=sCoreParams.core.stepPeriod  VariantControl=variantParams_FILTER_FIR_HIGHGAMMARIPPLE  mask(Bandpass Filter){}
      mask help: Design a bandpass filter
      settings: CopyFcn=fdesignblkfcn(gcbh, {'CopyFcn'});
      mask Help: helpview(mapfilelocation('dsp'), 'dspbandpassfilter');
      mask Display: disp('Bandpass');
  65-200Hz HighGammaRipple IIR : Subsystem  DialogController=fdesignblkfcn  InitFcn=fdesignblkfcn(gcbh, {'InitFcn'});  TreatAsAtomicUnit=on  SystemSampleTime=sCoreParams.core.stepPeriod  VariantControl=variantParams_FILTER_IIR_HIGHGAMMARIPPLE  mask(Bandpass Filter){}
      mask help: Design a bandpass filter
      settings: CopyFcn=fdesignblkfcn(gcbh, {'CopyFcn'});
      mask Help: helpview(mapfilelocation('dsp'), 'dspbandpassfilter');
      mask Display: disp('Bandpass');
  8-15Hz Alpha FIR : Subsystem  DialogController=fdesignblkfcn  InitFcn=fdesignblkfcn(gcbh, {'InitFcn'});  TreatAsAtomicUnit=on  SystemSampleTime=sCoreParams.core.stepPeriod  VariantControl=variantParams_FILTER_FIR_ALPHA  mask(Bandpass Filter){}
      mask help: Design a bandpass filter
      settings: CopyFcn=fdesignblkfcn(gcbh, {'CopyFcn'});
      mask Help: helpview(mapfilelocation('dsp'), 'dspbandpassfilter');
      mask Display: disp('Bandpass');
  8-15Hz Alpha IIR : Subsystem  DialogController=fdesignblkfcn  InitFcn=fdesignblkfcn(gcbh, {'InitFcn'});  TreatAsAtomicUnit=on  SystemSampleTime=sCoreParams.core.stepPeriod  VariantControl=variantParams_FILTER_IIR_ALPHA  mask(Bandpass Filter){}
      mask help: Design a bandpass filter
      settings: CopyFcn=fdesignblkfcn(gcbh, {'CopyFcn'});
      mask Help: helpview(mapfilelocation('dsp'), 'dspbandpassfilter');
      mask Display: disp('Bandpass');
  80-200Hz HFORipple FIR : Subsystem  DialogController=fdesignblkfcn  InitFcn=fdesignblkfcn(gcbh, {'InitFcn'});  TreatAsAtomicUnit=on  SystemSampleTime=sCoreParams.core.stepPeriod  VariantControl=variantParams_FILTER_FIR_HFORIPPLE  mask(Bandpass Filter){}
      mask help: Design a bandpass filter
      settings: CopyFcn=fdesignblkfcn(gcbh, {'CopyFcn'});
      mask Help: helpview(mapfilelocation('dsp'), 'dspbandpassfilter');
      mask Display: disp('Bandpass');
  80-200Hz HFORipple IIR : Subsystem  DialogController=fdesignblkfcn  InitFcn=fdesignblkfcn(gcbh, {'InitFcn'});  TreatAsAtomicUnit=on  SystemSampleTime=sCoreParams.core.stepPeriod  VariantControl=variantParams_FILTER_IIR_HFORIPPLE  mask(Bandpass Filter){}
      mask help: Design a bandpass filter
      settings: CopyFcn=fdesignblkfcn(gcbh, {'CopyFcn'});
      mask Help: helpview(mapfilelocation('dsp'), 'dspbandpassfilter');
      mask Display: disp('Bandpass');
  AllBand : Subsystem  TreatAsAtomicUnit=on  SystemSampleTime=sCoreParams.core.stepPeriod  VariantControl=variantParams_FILTER_ALLPASS
  VariableFreq FIR : Subsystem  TreatAsAtomicUnit=on  SystemSampleTime=sCoreParams.core.stepPeriod  VariantControl=variantParams_FILTER_FIR_EXTERNAL
  filteredData : Outport  SampleTime=sCoreParams.core.stepPeriod

== system ClosedLoopControl/Variant FEATURES/BandPower ==
  filteredData : Inport  SampleTime=sCoreParams.core.stepPeriod
  Mean : dspstat3/Mean  run=off  reset_popup=None  InputProcessing=Columns as channels (frame based)  directionMode=Each column  dimension=1  roiEnable=off  roiType=Rectangles  roiPortion=Entire ROI  roiOutput=Individual statistics for each ROI  roiFlag=off  outputDataTypeStr=Inherit: Same as accumulator  outputLastDataTypeStr=Inherit: Same as accumulator  outputMin=[]  outputMax=[]  roundingMode=Floor  overflowMode=off
  Product : Product
  RMS : dspstat3/RMS  Commented=on  run=off  directionMode=Each column  dimension=1  InputProcessing=Columns as channels (frame based)  reset_popup=None
  features : Outport  SampleTime=sCoreParams.core.stepPeriod
  wires:
  Product/1 -> Mean/1
  Mean/1 -> features/1
  filteredData/1 -> Product/1, Product/2

== system ClosedLoopControl/Variant FEATURES/BandPowerSmooth ==
  note: Poor hack  to have signals of nChan x nChan
      | The real feature is in the first column, the rest is all Zeros
      | (at some point change for variable size signals... )
  filteredData : Inport  SampleTime=sCoreParams.core.stepPeriod
  Buffer1 : Buffer  N=sCoreParams_Features_Data_SmoothWindowsDurationSamples  V=sCoreParams_Features_Data_SmoothWindowsDurationSamples-1  TreatMby1Signals=One channel
  Frame Conversion1 : FrameConversion  InheritSamplingMode=off  OutFrame=Sample-based
  Magnitude FFT : dspspect3/Magnitude FFT  Commented=on  mag_or_magsq=Magnitude squared  FFTImplementation=Auto  fftLenInherit=off  fftsize=sCoreParams.FrameSize  WrapInput=on
  Matrix Concatenate : Concatenate  Commented=on  Mode=Multidimensional array  ConcatenateDimension=2
  Mean1 : dspstat3/Mean  run=off  reset_popup=None  InputProcessing=Columns as channels (frame based)  directionMode=Each column  dimension=1  roiEnable=off  roiType=Rectangles  roiPortion=Entire ROI  roiOutput=Individual statistics for each ROI  roiFlag=off  outputDataTypeStr=Inherit: Same as accumulator  outputLastDataTypeStr=Inherit: Same as accumulator  outputMin=[]  outputMax=[]  roundingMode=Floor  overflowMode=off
  Mean2 : dspstat3/Mean  Commented=on  run=off  reset_popup=None  InputProcessing=Columns as channels (frame based)  directionMode=Each column  dimension=1  roiEnable=off  roiType=Rectangles  roiPortion=Entire ROI  roiOutput=Individual statistics for each ROI  roiFlag=off  outputDataTypeStr=Inherit: Same as accumulator  outputLastDataTypeStr=Inherit: Same as accumulator  outputMin=[]  outputMax=[]  roundingMode=Floor  overflowMode=off
  RMS : dspstat3/RMS  run=off  directionMode=Each column  dimension=1  InputProcessing=Columns as channels (frame based)  reset_popup=None
  ZEROS : Constant  Commented=on  Value=zeros(sCoreParams_decoders_txDetector_nChannels, sCoreParams_decoders_txDetector_nChannels-1)  VectorParams1D=off
  features : Outport  SampleTime=sCoreParams.core.stepPeriod
  wires:
  Buffer1/1 -> Mean1/1
  RMS/1 -> Buffer1/1
  filteredData/1 -> RMS/1
  Magnitude FFT/1 -> Mean2/1
  Mean1/1 -> Frame Conversion1/1
  Frame Conversion1/1 -> features/1
  ZEROS/1 -> Matrix Concatenate/2

== system ClosedLoopControl/Variant FEATURES/Correlation ==
  filteredData : Inport  SampleTime=sCoreParams.core.stepPeriod
  Buffer1 : Buffer  N=sCoreParams.Features.Coherence.WindowDurationSamples  V=sCoreParams.Features.Coherence.WindowDurationSamples - sCoreParams.FrameSize  TreatMby1Signals=One channel
  xCorrCoef : MATLAB Function  TreatAsAtomicUnit=on
  features : Outport  SampleTime=sCoreParams.core.stepPeriod
  wires:
  xCorrCoef/1(rxy) -> features/1
  filteredData/1 -> Buffer1/1
  Buffer1/1 -> xCorrCoef/1(filteredData)

== system ClosedLoopControl/Variant FEATURES/Variance ==
  filteredData : Inport  SampleTime=sCoreParams.core.stepPeriod
  Variance : dspstat3/Variance  run=off  reset_popup=None  InputProcessing=Columns as channels (frame based)  directionMode=Each column  dimension=1  roiEnable=off  roiType=Rectangles  roiPortion=Entire ROI  roiOutput=Individual statistics for each ROI  roiFlag=off  roundingMode=Floor  overflowMode=off
  features : Outport  SampleTime=sCoreParams.core.stepPeriod
  wires:
  Variance/1 -> features/1
  filteredData/1 -> Variance/1

== system ClosedLoopControl/Variant FEATURES/VarianceOfPower ==
  filteredData : Inport  SampleTime=sCoreParams.core.stepPeriod
  Magnitude FFT : dspspect3/Magnitude FFT  mag_or_magsq=Magnitude squared  FFTImplementation=Auto  fftLenInherit=off  fftsize=32  WrapInput=on
  Mean : dspstat3/Mean  run=off  reset_popup=None  InputProcessing=Columns as channels (frame based)  directionMode=Each column  dimension=1  roiEnable=off  roiType=Rectangles  roiPortion=Entire ROI  roiOutput=Individual statistics for each ROI  roiFlag=off  outputDataTypeStr=Inherit: Same as accumulator  outputLastDataTypeStr=Inherit: Same as accumulator  outputMin=[]  outputMax=[]  roundingMode=Floor  overflowMode=off
  Variance : dspstat3/Variance  run=off  reset_popup=None  InputProcessing=Columns as channels (frame based)  directionMode=Each column  dimension=1  roiEnable=off  roiType=Rectangles  roiPortion=Entire ROI  roiOutput=Individual statistics for each ROI  roiFlag=off  roundingMode=Floor  overflowMode=off
  features : Outport  SampleTime=sCoreParams.core.stepPeriod
  wires:
  filteredData/1 -> Magnitude FFT/1
  Magnitude FFT/1 -> Variance/1
  Variance/1 -> Mean/1
  Mean/1 -> features/1

== system ClosedLoopControl/Variant THRESHOLDS/BandPower ==
  filteredData : Inport  SampleTime=sCoreParams.core.stepPeriod
  Trigger : Inport  Port=2  SampleTime=sCoreParams.core.stepPeriod
  PassIfTrue : Inport  Port=3  SampleTime=sCoreParams.core.stepPeriod
  PreviousThreshold : Inport  Port=4  SampleTime=sCoreParams.core.stepPeriod
  Magnitude FFT : dspspect3/Magnitude FFT  mag_or_magsq=Magnitude squared  FFTImplementation=Auto  fftLenInherit=on  fftsize=32  WrapInput=on
  Mean : dspstat3/Mean  run=off  reset_popup=None  InputProcessing=Columns as channels (frame based)  directionMode=Each column  dimension=1  roiEnable=off  roiType=Rectangles  roiPortion=Entire ROI  roiOutput=Individual statistics for each ROI  roiFlag=off  outputDataTypeStr=Inherit: Same as accumulator  outputLastDataTypeStr=Inherit: Same as accumulator  outputMin=[]  outputMax=[]  roundingMode=Floor  overflowMode=off
  Switch : Switch  Criteria=u2 > Threshold  InputSameDT=on
  thFeatures : Outport  SampleTime=sCoreParams.core.stepPeriod
  IsUpdatingThresh : Outport  Port=2  SampleTime=sCoreParams.core.stepPeriod
  wires:
  filteredData/1 -> Magnitude FFT/1
  Magnitude FFT/1 -> Mean/1
  PassIfTrue/1 -> IsUpdatingThresh/1
  PreviousThreshold/1 -> Switch/3
  Switch/1 -> thFeatures/1
  Trigger/1 -> Switch/2
  Mean/1 -> Switch/1

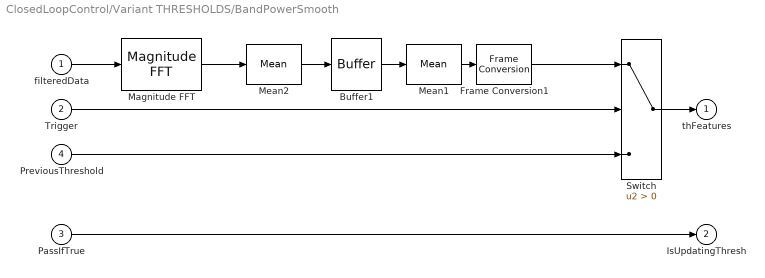
== system ClosedLoopControl/Variant THRESHOLDS/BandPowerSmooth ==
  filteredData : Inport  SampleTime=sCoreParams.core.stepPeriod
  Trigger : Inport  Port=2  SampleTime=sCoreParams.core.stepPeriod
  PassIfTrue : Inport  Port=3  SampleTime=sCoreParams.core.stepPeriod
  PreviousThreshold : Inport  Port=4  SampleTime=sCoreParams.core.stepPeriod
  Buffer1 : Buffer  N=sCoreParams.Features.Baseline.SmoothWindowsDurationSamples  V=sCoreParams.Features.Baseline.SmoothWindowsDurationSamples-1  TreatMby1Signals=One channel
  Frame Conversion1 : FrameConversion  InheritSamplingMode=off  OutFrame=Sample-based
  Magnitude FFT : dspspect3/Magnitude FFT  mag_or_magsq=Magnitude squared  FFTImplementation=Auto  fftLenInherit=on  fftsize=32  WrapInput=on
  Mean1 : dspstat3/Mean  run=off  reset_popup=None  InputProcessing=Columns as channels (frame based)  directionMode=Each column  dimension=1  roiEnable=off  roiType=Rectangles  roiPortion=Entire ROI  roiOutput=Individual statistics for each ROI  roiFlag=off  outputDataTypeStr=Inherit: Same as accumulator  outputLastDataTypeStr=Inherit: Same as accumulator  outputMin=[]  outputMax=[]  roundingMode=Floor  overflowMode=off
  Mean2 : dspstat3/Mean  run=off  reset_popup=None  InputProcessing=Columns as channels (frame based)  directionMode=Each column  dimension=1  roiEnable=off  roiType=Rectangles  roiPortion=Entire ROI  roiOutput=Individual statistics for each ROI  roiFlag=off  outputDataTypeStr=Inherit: Same as accumulator  outputLastDataTypeStr=Inherit: Same as accumulator  outputMin=[]  outputMax=[]  roundingMode=Floor  overflowMode=off
  Switch : Switch  Criteria=u2 > Threshold  InputSameDT=on
  thFeatures : Outport  SampleTime=sCoreParams.core.stepPeriod
  IsUpdatingThresh : Outport  Port=2  SampleTime=sCoreParams.core.stepPeriod
  wires:
  filteredData/1 -> Magnitude FFT/1
  Buffer1/1 -> Mean1/1
  Mean1/1 -> Frame Conversion1/1
  PassIfTrue/1 -> IsUpdatingThresh/1
  PreviousThreshold/1 -> Switch/3
  Switch/1 -> thFeatures/1
  Trigger/1 -> Switch/2
  Magnitude FFT/1 -> Mean2/1
  Frame Conversion1/1 -> Switch/1
  Mean2/1 -> Buffer1/1

== system ClosedLoopControl/Variant THRESHOLDS/Variance ==
  filteredData : Inport  SampleTime=sCoreParams.core.stepPeriod
  Trigger : Inport  Port=2  SampleTime=sCoreParams.core.stepPeriod
  PassIfTrue : Inport  Port=3  SampleTime=sCoreParams.core.stepPeriod
  PreviousThreshold : Inport  Port=4  SampleTime=sCoreParams.core.stepPeriod
  Switch : Switch  Criteria=u2 > Threshold  InputSameDT=on
  Variance : dspstat3/Variance  run=off  reset_popup=None  InputProcessing=Columns as channels (frame based)  directionMode=Each column  dimension=1  roiEnable=off  roiType=Rectangles  roiPortion=Entire ROI  roiOutput=Individual statistics for each ROI  roiFlag=off  roundingMode=Floor  overflowMode=off
  thFeatures : Outport  SampleTime=sCoreParams.core.stepPeriod
  IsUpdatingThresh : Outport  Port=2  SampleTime=sCoreParams.core.stepPeriod
  wires:
  filteredData/1 -> Variance/1
  PassIfTrue/1 -> IsUpdatingThresh/1
  PreviousThreshold/1 -> Switch/3
  Switch/1 -> thFeatures/1
  Trigger/1 -> Switch/2
  Variance/1 -> Switch/1

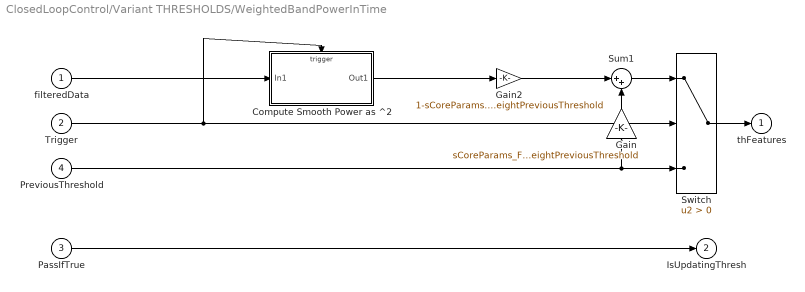
== system ClosedLoopControl/Variant THRESHOLDS/WeightedBandPowerInTime ==
  filteredData : Inport  SampleTime=sCoreParams.core.stepPeriod
  Trigger : Inport  Port=2  SampleTime=sCoreParams.core.stepPeriod
  PassIfTrue : Inport  Port=3  SampleTime=sCoreParams.core.stepPeriod
  PreviousThreshold : Inport  Port=4  SampleTime=sCoreParams.core.stepPeriod
  Compute Smooth Power as ^2 : Subsystem
  Gain : Gain  Gain=sCoreParams_Features_Baseline_weightPreviousThreshold  OutDataTypeStr=Inherit: Same as input
  Gain2 : Gain  Gain=1-sCoreParams.Features.Baseline.weightPreviousThreshold
  Sum1 : Sum  Inputs=|++
  Switch : Switch  Criteria=u2 > Threshold  InputSameDT=on
  thFeatures : Outport  SampleTime=sCoreParams.core.stepPeriod
  IsUpdatingThresh : Outport  Port=2  SampleTime=sCoreParams.core.stepPeriod
  wires:
  PassIfTrue/1 -> IsUpdatingThresh/1
  Trigger/1 -> Compute Smooth Power as ^2/Trigger, Switch/2
  Sum1/1 -> Switch/1
  Gain/1 -> Sum1/2
  Switch/1 -> thFeatures/1
  PreviousThreshold/1 -> Gain/1, Switch/3
  filteredData/1 -> Compute Smooth Power as ^2/1(In1)
  Compute Smooth Power as ^2/1(Out1) -> Gain2/1
  Gain2/1 -> Sum1/1

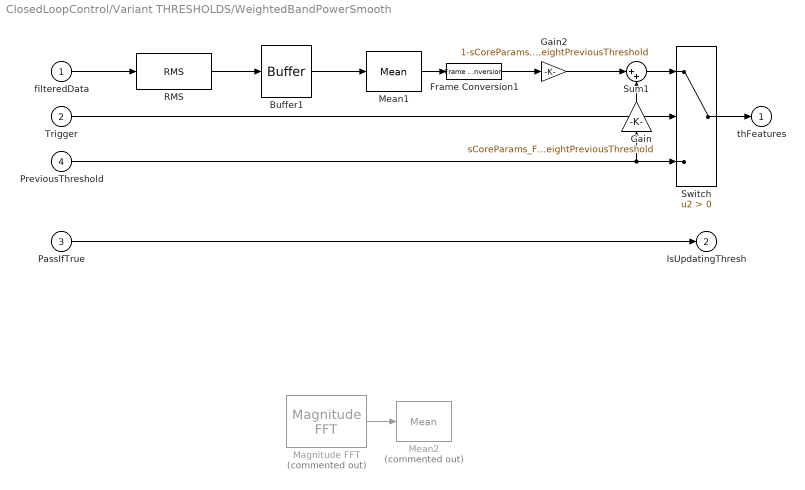
== system ClosedLoopControl/Variant THRESHOLDS/WeightedBandPowerSmooth ==
  filteredData : Inport  PortDimensions=[sCoreParams.Features.Baseline.durationSamples sCoreParams.decoders.txDetector.nFeatures]  SampleTime=sCoreParams.core.stepPeriod
  Trigger : Inport  Port=2  SampleTime=sCoreParams.core.stepPeriod
  PassIfTrue : Inport  Port=3  SampleTime=sCoreParams.core.stepPeriod
  PreviousThreshold : Inport  Port=4  PortDimensions=[1 sCoreParams.decoders.txDetector.nFeatures]  SampleTime=sCoreParams.core.stepPeriod
  Buffer1 : Buffer  N=sCoreParams.Features.Baseline.SmoothWindowsDurationSamples  V=sCoreParams.Features.Baseline.SmoothWindowsDurationSamples-1  TreatMby1Signals=One channel
  Frame Conversion1 : FrameConversion  InheritSamplingMode=off  OutFrame=Sample-based
  Gain : Gain  Gain=sCoreParams_Features_Baseline_weightPreviousThreshold  OutDataTypeStr=Inherit: Same as input
  Gain2 : Gain  Gain=1-sCoreParams.Features.Baseline.weightPreviousThreshold
  Magnitude FFT : dspspect3/Magnitude FFT  Commented=on  mag_or_magsq=Magnitude squared  FFTImplementation=Auto  fftLenInherit=off  fftsize=sCoreParams.Features.Baseline.durationSamples  WrapInput=on
  Mean1 : dspstat3/Mean  run=off  reset_popup=None  InputProcessing=Columns as channels (frame based)  directionMode=Each column  dimension=1  roiEnable=off  roiType=Rectangles  roiPortion=Entire ROI  roiOutput=Individual statistics for each ROI  roiFlag=off  outputDataTypeStr=Inherit: Same as accumulator  outputLastDataTypeStr=Inherit: Same as accumulator  outputMin=[]  outputMax=[]  roundingMode=Floor  overflowMode=off
  Mean2 : dspstat3/Mean  Commented=on  run=off  reset_popup=None  InputProcessing=Columns as channels (frame based)  directionMode=Each column  dimension=1  roiEnable=off  roiType=Rectangles  roiPortion=Entire ROI  roiOutput=Individual statistics for each ROI  roiFlag=off  outputDataTypeStr=Inherit: Same as accumulator  outputLastDataTypeStr=Inherit: Same as accumulator  outputMin=[]  outputMax=[]  roundingMode=Floor  overflowMode=off
  RMS : dspstat3/RMS  run=off  directionMode=Each column  dimension=1  InputProcessing=Columns as channels (frame based)  reset_popup=None
  Sum1 : Sum  Inputs=|++
  Switch : Switch  Criteria=u2 > Threshold  InputSameDT=on
  thFeatures : Outport  PortDimensions=[1 sCoreParams.decoders.txDetector.nFeatures]  SampleTime=sCoreParams.core.stepPeriod
  IsUpdatingThresh : Outport  Port=2  SampleTime=sCoreParams.core.stepPeriod
  wires:
  PassIfTrue/1 -> IsUpdatingThresh/1
  Trigger/1 -> Switch/2
  Sum1/1 -> Switch/1
  Gain/1 -> Sum1/2
  Magnitude FFT/1 -> Mean2/1
  PreviousThreshold/1 -> Gain/1, Switch/3
  Switch/1 -> thFeatures/1
  Gain2/1 -> Sum1/1
  RMS/1 -> Buffer1/1
  Mean1/1 -> Frame Conversion1/1
  Buffer1/1 -> Mean1/1
  filteredData/1 -> RMS/1
  Frame Conversion1/1 -> Gain2/1
